simulink model "ex_inverter_single_full_bridge_unipoPWM"  (R2022b)
settings: Solver=VariableStepAuto  StartTime=0.0  StopTime=0.1  RelTol=1e-3
libraries: spsMosfetLib x4, spsFourierLib x3, spsVoltageMeasurementLib x2, spsDCVoltageSourceLib x2, spsGroundLib x1, spsMultimeterLib x1, spsRMSLib x1, simulink x1, spsSeriesRLCBranchLib x1, spsTHDLib x1, sps_lib x1
settings Model: Creator=realj  LastModifiedBy=realj

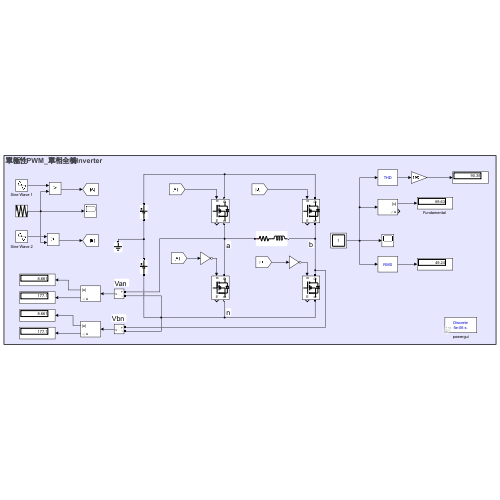
[thumbnail: Simulink's stored preview of the top-level diagram]
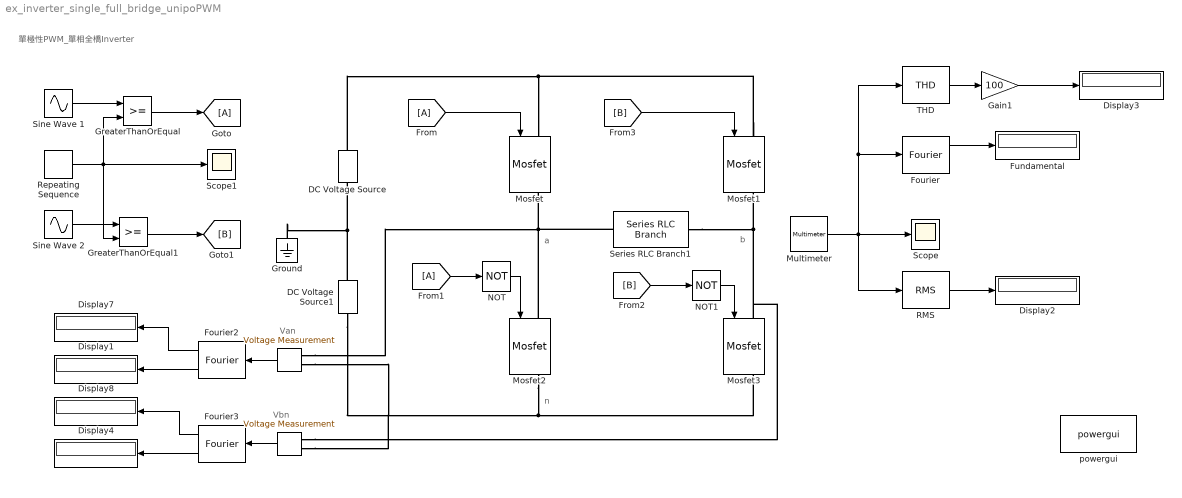
== system ex_inverter_single_full_bridge_unipoPWM ==
  note: a
  note: 單極性PWM_單相全橋Inverter
  note: b
  note: n
  note: Van
  note: Vbn
  " " : spsVoltageMeasurementLib/Voltage Measurement  PhasorSimulation=off  OutputType=Complex  PSBequivalent=0
  "  " : spsVoltageMeasurementLib/Voltage Measurement  PhasorSimulation=off  OutputType=Complex  PSBequivalent=0
  DC Voltage Source : spsDCVoltageSourceLib/DC Voltage Source  Amplitude=50  Measurements=None
  DC Voltage Source1 : spsDCVoltageSourceLib/DC Voltage Source  Amplitude=50  Measurements=None
  Display{1..4,7..8} (6 alike) : Display
  Fourier : spsFourierLib/Fourier  Freq=50  n=1  InInit=[0, 0]  Ts=0
  Fourier2 : spsFourierLib/Fourier  Freq=50  n=26  InInit=[0, 0]  Ts=0
  Fourier3 : spsFourierLib/Fourier  Freq=50  n=26  InInit=[0, 0]  Ts=0
  From : From
  From1 : From
  "Fundamental " : Display
  Gain1 : Gain  Gain=100
  Goto : Goto
  GreaterThanOrEqual : RelationalOperator  OutDataTypeStr=boolean  RndMeth=Simplest  InputSameDT=off
  GreaterThanOrEqual1 : RelationalOperator  OutDataTypeStr=boolean  RndMeth=Simplest  InputSameDT=off
  Ground : spsGroundLib/Ground  LConnTagsString=a
  Mosfet{,1..3} (4 alike) : spsMosfetLib/Mosfet  Ron=0.1  Lon=0  Rd=0.01  Vfd=0  IC=0  Rs=1e5  Cs=inf  Measurements=on
  Multimeter : spsMultimeterLib/Multimeter  L=1  sel=1  yselected={}  Gain=1  OutputType=Complex  PlotAtSimulationStop=off  PhasorSimulation=off
  NOT : Logic  Operator=NOT  IconShape=distinctive  AllPortsSameDT=off  OutDataTypeStr=boolean
  NOT1 : Logic  Operator=NOT  IconShape=distinctive  AllPortsSameDT=off  OutDataTypeStr=boolean
  RMS : spsRMSLib/RMS  TrueRMS=off  Freq=50  RMSInit=0  Ts=0
  Repeating Sequence : simulink/Sources/Repeating Sequence  rep_seq_t=[0 1 2 3 4]*1/(24*50*4)  rep_seq_y=[0 1 0 -1 0]
  Scope : Scope
  Scope1 : Scope
  Series RLC Branch1 : spsSeriesRLCBranchLib/Series RLC Branch  LConnTagsString=__new0  RConnTagsString=__new0  BranchType=RL  Resistance=25  Inductance=1e-3  SetiL0=off  InitialCurrent=0  Capacitance=1e-6  Setx0=off  InitialVoltage=0  Measurements=Branch voltage
  Sine Wave 1 : Sin  Amplitude=.7  Frequency=2*pi*50  SampleTime=0
  Sine Wave 2 : Sin  Amplitude=.7  Frequency=2*pi*50  Phase=pi  SampleTime=0
  THD : spsTHDLib/THD  Freq=50  Ts=0
  powergui : sps_lib/powergui  Priority=1  SimulationMode=Discrete  SampleTime=5e-6  frequency=60  Iterations=50  frequencyindice=0  Pbase=100e6  ErrMax=1e-4  UnitsV=kV  UnitsW=MW  buscounter=0  FunctionMessages=off  echomessages=off  EnableUseOfTLC=off  CurrentSourceSwitches=off  DisableSnubberDevices=off  DisableRonSwitches=off  DisableVfSwitches=off  DisplayEquations=off  AutomaticDiscreteSolvers=off  SolverType=Tustin/Backward Euler (TBE)  Interpol=off  ExternalGateDelay=off  methode=off  Ts=100  x0status=blocks  SPID=on  SwTol=0  HookPort=off  NonlinearTolerance=1e-4  nMaxIteration=100  ContinueOnMaxIteration=off  RestoreLinks=warning  ResistiveCurrentMeasurement=off  Frange=[0:2:500]  Ylog=off  Xlog=on  ShowGrid=off  save=off  variable=ZData  structure=0  ZoomFFT=off  StartTime=0.0  cycles=1  DisplayStyle=1  fundamental=60  FreqAxis=off  MaxFrequency=1000  frequencyindicesteady=1  RmsSteady=1  display=off
  wires:
  Sine Wave 1/1 -> GreaterThanOrEqual/1
  Repeating Sequence/1 -> GreaterThanOrEqual1/2, Scope1/1, GreaterThanOrEqual/2
  Sine Wave 2/1 -> GreaterThanOrEqual1/1
  GreaterThanOrEqual/1 -> Goto/1
  GreaterThanOrEqual1/1 -> [B]
  From/1 -> Mosfet/1
  From1/1 -> NOT/1
  NOT/1 -> Mosfet2/1
  NOT1/1 -> Mosfet3/1
  [B] -> NOT1/1
  [B] -> Mosfet1/1
  RMS/1 -> Display2/1
  Fourier/1 -> "Fundamental "/1
  THD/1 -> Gain1/1
  Multimeter/1 -> RMS/1, Fourier/1, THD/1, Scope/1
  " "/1 -> Fourier2/1
  "  "/1 -> Fourier3/1
  Gain1/1 -> Display3/1
  Fourier2/1 -> Display7/1
  Fourier3/1 -> Display8/1
  Fourier2/2 -> Display1/1
  Fourier3/2 -> Display4/1
  connections:
  Series RLC Branch1/RConn1 -- "  "/LConn1 -- Mosfet3/LConn1 -- Mosfet1/RConn1
  Series RLC Branch1/LConn1 -- Mosfet/RConn1 -- " "/LConn1 -- Mosfet2/LConn1
  DC Voltage Source/RConn1 -- Mosfet1/LConn1 -- Mosfet/LConn1
  Mosfet2/RConn1 -- "  "/LConn2 -- " "/LConn2 -- DC Voltage Source1/LConn1 -- Mosfet3/RConn1
  DC Voltage Source1/RConn1 -- Ground/LConn1 -- DC Voltage Source/LConn1
